simulink model "Solution_of_the_SE_Simulink"  (R2023a)
settings: Solver=VariableStepAuto  StartTime=0.0  StopTime=10.0  RelTol=1e-3
values from neighbouring files (symbols this model uses):
  A = [0 1; -2 -3]    [Solution_of_the_SE.m]    (also in sim1.m)
  B = [0; 1]    [Solution_of_the_SE.m]    (also in sim1.m)
  C = [1 1]    [Solution_of_the_SE.m]    (also in sim1.m)
  x_init = [x_1(i); x_2(i)]    [Solution_of_the_SE.m]    (also in sim1.m)
settings Model: Creator=m260477  LastModifiedBy=m260477

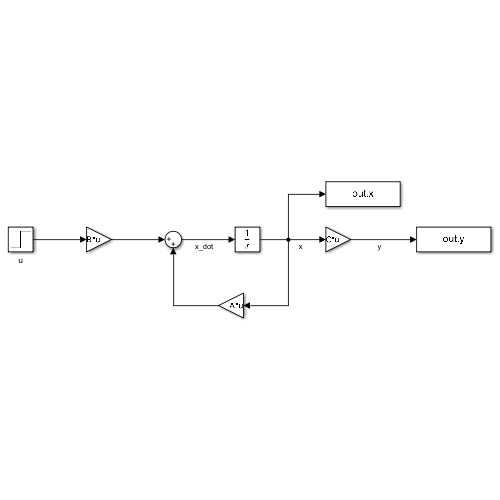
[thumbnail: Simulink's stored preview of the top-level diagram]
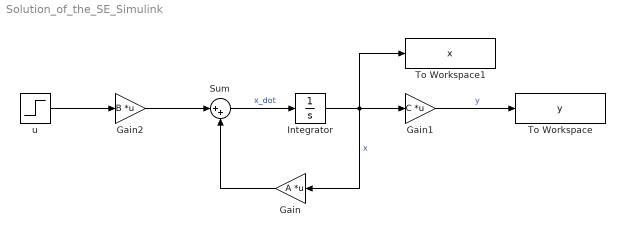
== system Solution_of_the_SE_Simulink ==
  Gain : Gain  Gain=A  Multiplication=Matrix(K*u)
  Gain1 : Gain  Gain=C  Multiplication=Matrix(K*u)
  Gain2 : Gain  Gain=B  Multiplication=Matrix(K*u)
  Integrator : Integrator  InitialCondition=x_init
  Sum : Sum  Inputs=|++
  To Workspace : ToWorkspace  VariableName=y  SaveFormat=Timeseries  SampleTime=-1
  To Workspace1 : ToWorkspace  VariableName=x  SaveFormat=Timeseries  SampleTime=-1
  u : Step  Time=0  After=u  SampleTime=0
  wires:
  Integrator/1 -> To Workspace1/1, Gain1/1, Gain/1  "x"
  Gain1/1 -> To Workspace/1  "y"
  Sum/1 -> Integrator/1  "x_dot"
  Gain/1 -> Sum/2
  Gain2/1 -> Sum/1
  u/1 -> Gain2/1
